simulink model "Dynamics_Model"  (R2024b)
settings: Solver=VariableStepAuto  StartTime=0.0  StopTime=10.0  RelTol=1e-3
undefined symbols (not defined in the file or in its folder): DiscIntNeverNeededParam
libraries: simulink x2
settings Model: Creator=himma  LastModifiedBy=himma

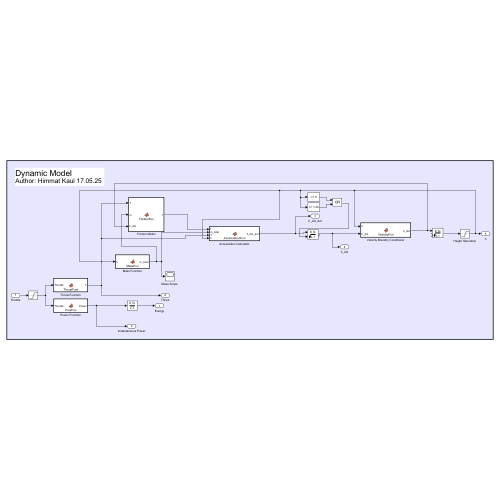
[thumbnail: Simulink's stored preview of the top-level diagram]
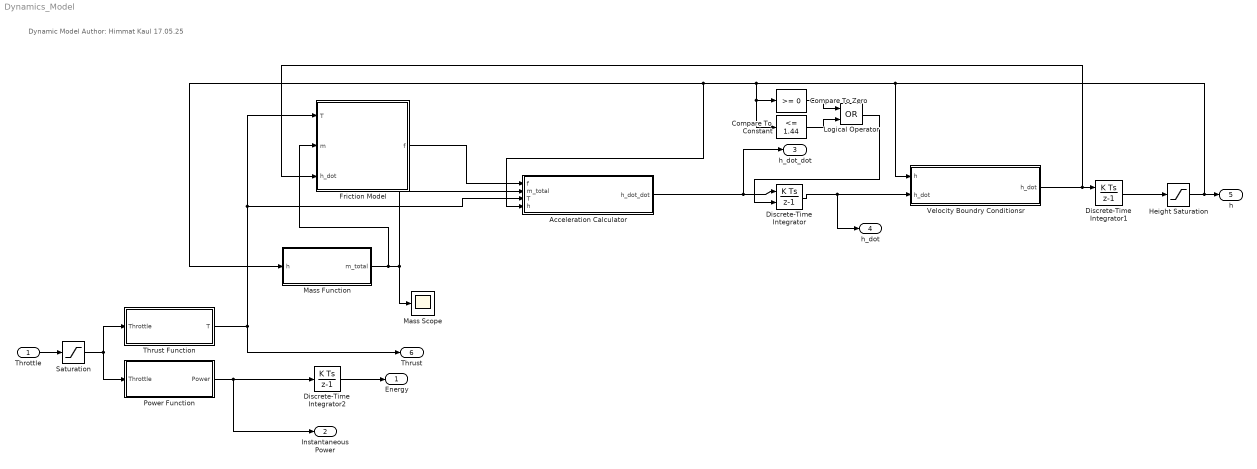
== system Dynamics_Model ==
  note: Dynamic Model
      | Author: Himmat Kaul 17.05.25
  Throttle : Inport
  Acceleration Calculator : MATLAB Function  TreatAsAtomicUnit=on
  Compare To Constant : simulink/Logic and Bit Operations/Compare To Constant  relop=<=  const=1.44  OutDataTypeStr=boolean
  Compare To Zero : simulink/Logic and Bit Operations/Compare To Zero  relop=>=  OutDataTypeStr=boolean
  Discrete-Time Integrator : DiscreteIntegrator  ExternalReset=rising  SampleTime=-1  ICPrevOutput=DiscIntNeverNeededParam  ICPrevScaledInput=DiscIntNeverNeededParam
  Discrete-Time Integrator1 : DiscreteIntegrator  ExternalReset=rising  SampleTime=-1  ICPrevOutput=DiscIntNeverNeededParam  ICPrevScaledInput=DiscIntNeverNeededParam
  Discrete-Time Integrator2 : DiscreteIntegrator  SampleTime=-1  ICPrevOutput=DiscIntNeverNeededParam  ICPrevScaledInput=DiscIntNeverNeededParam
  Friction Model : MATLAB Function  TreatAsAtomicUnit=on
  Height Saturation : Saturate  UpperLimit=1.44  LowerLimit=0
  Logical Operator : Logic  Operator=OR  AllPortsSameDT=off  OutDataTypeStr=boolean
  Mass Function : MATLAB Function  TreatAsAtomicUnit=on
  Mass Scope : Scope
  Power Function : MATLAB Function  TreatAsAtomicUnit=on
  Saturation : Saturate  UpperLimit=0.6  LowerLimit=0
  Thrust Function : MATLAB Function  TreatAsAtomicUnit=on
  Velocity Boundry Conditionsr : MATLAB Function  TreatAsAtomicUnit=on
  Energy : Outport
  Instantaneous Power : Outport  Port=2
  h_dot_dot : Outport  Port=3
  h_dot : Outport  Port=4
  h : Outport  Port=5
  Thrust : Outport  Port=6
  wires:
  Throttle/1 -> Saturation/1
  Thrust Function/1(T) -> Friction Model/1(T), Acceleration Calculator/3(T), Thrust/1
  Power Function/1(Power) -> Discrete-Time Integrator2/1, Instantaneous Power/1
  Mass Function/1(m_total) -> Friction Model/2(m), Mass Scope/1, Acceleration Calculator/2(m_total)
  Acceleration Calculator/1(h_dot_dot) -> Discrete-Time Integrator/1, h_dot_dot/1
  Friction Model/1(f) -> Acceleration Calculator/1(f)
  Discrete-Time Integrator/1 -> Velocity Boundry Conditionsr/2("h_dot "), h_dot/1
  Discrete-Time Integrator1/1 -> Height Saturation/1
  Discrete-Time Integrator2/1 -> Energy/1
  Saturation/1 -> Power Function/1(Throttle), Thrust Function/1(Throttle)
  Velocity Boundry Conditionsr/1(h_dot) -> Friction Model/3(h_dot), Discrete-Time Integrator1/1
  Compare To Zero/1 -> Logical Operator/1
  Compare To Constant/1 -> Logical Operator/2
  Height Saturation/1 -> Velocity Boundry Conditionsr/1(h), Compare To Constant/1, Compare To Zero/1, Acceleration Calculator/4(h), Mass Function/1(h), h/1
  Logical Operator/1 -> Discrete-Time Integrator/2

== matlab function Dynamics_Model/Thrust Function ==
  data: Throttle input; T output
function T = ThrustFunt(Throttle)

% 
% a =    2.186e+05;  
% b =     -0.08123;  
% c =   -2.186e+05;  
% d =      -0.0813;
% 
% T = 2 * (a*exp(b*Throttle) + c*exp(d*Throttle));

T = 2 * 15 * Throttle;

== matlab function Dynamics_Model/Power Function ==
  data: Throttle input; Power output
function Power = PowFun(Throttle)

a =   3.418e+06;  
b =       0.179;  
c =  -3.418e+06;  
d =      0.1789;

Power = 2 * (a*exp(b*Throttle) + c*exp(d*Throttle));

== matlab function Dynamics_Model/Friction Model ==
  data: f output; T input; m input; h_dot input
function f = FrictionFun(T, m, h_dot)

% Physical parameters
g = 9.81;
% f_static = 0.0013*g; %% given..
mu_d = 0.17; %% 0.17 upper bound

% Geometry Parameters
l_t = 0.01;
l_cg = 0.01;
L_c = 0.01;

%Piecewise friction function

if h_dot == 0 %% make range

    f = 0.26 * g;

    % if (abs(T-m*g) > 2*f_static)      
    %     f = T - m*g;
    % else
    %     f = 2*f_static;
    % end
else 
    % Calculate Normal Force
    N = (T * l_t - m*g*l_cg)/L_c;

    f = mu_d * abs(N) * sign(h_dot);
end    

% 
% f = 0;

== matlab function Dynamics_Model/Velocity Boundry Conditionsr ==
  data: h input; h_dot input; h_dot output
function h_dot = VelocityFun(h, h_dot)


% if (h == 0) && (h < 0) 
%     h_dot = 0;
% elseif (h == 1.44) && (h > 0) 
%     h_dot = 0;
% else
    h_dot = h_dot;
% end

== matlab function Dynamics_Model/Acceleration Calculator ==
  data: f input; h_dot_dot output; m_total input; T input; h input
function h_dot_dot = AccelerationFun(f, m_total, T, h)

g = 9.81;

m_intertial = m_total + 0.328 + 0.8;

h_dot_dot = (T - f - m_total * g) / m_intertial ;
 
if (h_dot_dot < 0) && (h == 0)
    h_dot_dot = 0;
end

if (h_dot_dot > 0) && (h == 1.44)
    h_dot_dot = 0;
end

== matlab function Dynamics_Model/Mass Function ==
  data: h input; m_total output
function m_total = MassFun(h)
 
m_copter = 0.05; % kg
m_electronics = 1.51*2/9.81; % kg 
m_cart = 0.15; %kg
m_cable = 2 * (0.095 * h + 0.0532); % kg

% if case for caternary stufff....




m_total = m_cart + m_copter + m_electronics + m_cable;

% m_total =;
